simulink model "nav_test"  (R2020a)
settings: Solver=FixedStepAuto  StartTime=0.0  StopTime=500  FixedStep=1  RelTol=1e-3
settings Model: Creator=joaoc  LastModifiedBy=joaoc

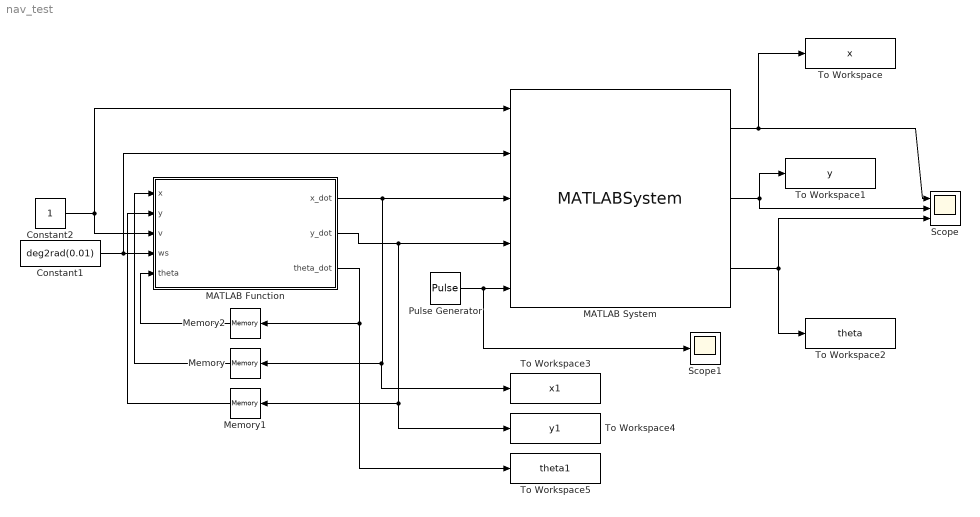
== system nav_test ==
  Constant1 : Constant  Value=deg2rad(0.01)
  Constant2 : Constant
  MATLAB Function : MATLAB Function  TreatAsAtomicUnit=on
  MATLAB System : MATLABSystem  System=navigation  initial_x=0  initial_y=0  initial_theta=0  q_gain=0.001  r_gain=0.5  SimulateUsing=Code generation
      mask Type: navigation
      mask Display:
      | disp('navigation');
      | port_label('input',1,'V');
      | port_label('input',2,'omega_s');
      | port_label('input',3,'x_real');
      | port_label('input',4,'y_real');
      | port_label('input',5,'GPS');
      | port_label('output',1,'x');
      | port_label('output',2,'y');
      | port_label('output',3,'theta');
  Memory : Memory
  Memory1 : Memory
  Memory2 : Memory
  Pulse Generator : DiscretePulseGenerator  PulseType=Time based  Period=300  PulseWidth=50  PhaseDelay=50
  Scope : Scope  NumInputPorts=3
  Scope1 : Scope
  To Workspace : ToWorkspace  VariableName=x  SampleTime=-1
      settings: Save2DSignal=2-D array (concatenate along first dimension)
  To Workspace1 : ToWorkspace  VariableName=y  SampleTime=-1
      settings: Save2DSignal=2-D array (concatenate along first dimension)
  To Workspace2 : ToWorkspace  VariableName=theta  SampleTime=-1
      settings: Save2DSignal=2-D array (concatenate along first dimension)
  To Workspace3 : ToWorkspace  VariableName=x1  SampleTime=-1
      settings: Save2DSignal=2-D array (concatenate along first dimension)
  To Workspace4 : ToWorkspace  VariableName=y1  SampleTime=-1
      settings: Save2DSignal=2-D array (concatenate along first dimension)
  To Workspace5 : ToWorkspace  VariableName=theta1  SampleTime=-1
      settings: Save2DSignal=2-D array (concatenate along first dimension)
  wires:
  Constant1/1 -> MATLAB System/2, MATLAB Function/4(ws)
  Constant2/1 -> MATLAB System/1, MATLAB Function/3(v)
  MATLAB System/1 -> To Workspace/1, Scope/1
  MATLAB System/2 -> To Workspace1/1, Scope/2
  MATLAB System/3 -> To Workspace2/1, Scope/3
  MATLAB Function/2(y_dot) -> To Workspace4/1, Memory1/1, MATLAB System/4
  MATLAB Function/1(x_dot) -> To Workspace3/1, Memory/1, MATLAB System/3
  Memory/1 -> MATLAB Function/1(x)
  Memory1/1 -> MATLAB Function/2(y)
  MATLAB Function/3(theta_dot) -> To Workspace5/1, Memory2/1
  Memory2/1 -> MATLAB Function/5(theta)
  Pulse Generator/1 -> Scope1/1, MATLAB System/5

== matlab function nav_test/MATLAB Function ==
  data: x input; x_dot output; y input; v input; ws input; theta input; y_dot output; theta_dot output
function [x_dot, y_dot, theta_dot] = model_ss(x,y,v,ws,theta)
    
    A = eye(3);
    B = [cos(theta), 0; sin(theta), 0; 0, 1];
    u_vec = [v; ws];
    state = [x; y; theta];    
    
    state = A*state + B*u_vec;
    
    x_dot=state(1);
    y_dot=state(2);
    theta_dot=state(3);
    
end
